simulink library "TriadActivation_lib"  (R2018b)
settings: Solver=VariableStepAuto  StartTime=0.0  StopTime=10.0  RelTol=1e-3
undefined symbols (not defined in the file): fswParams
libraries: dspswit3 x1
settings Model: Creator=kylle  LastModifiedBy=kylle

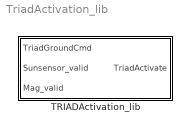
== system TriadActivation_lib ==
  TRIADActivation_lib : Subsystem  TreatAsAtomicUnit=on
      settings: RTWFcnNameOpts=Use subsystem name  RTWFileNameOpts=Use subsystem name

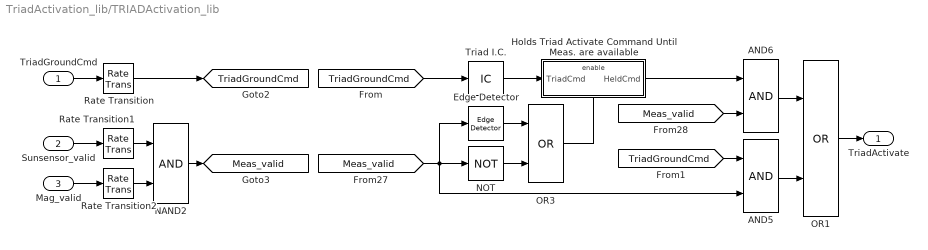
== system TriadActivation_lib/TRIADActivation_lib ==
  TriadGroundCmd : Inport
  Sunsensor_valid : Inport  Port=2
  Mag_valid : Inport  Port=3
  AND5 : Logic  AllPortsSameDT=off  OutDataTypeStr=boolean
  AND6 : Logic  AllPortsSameDT=off  OutDataTypeStr=boolean
  Edge Detector : dspswit3/Edge Detector  InputProcessing=Columns as channels (frame based)
      settings: SourceProductName=DSP System Toolbox  SourceProductBaseCode=DS
  Holds Triad Activate Command Until Meas. are available : Subsystem  TreatAsAtomicUnit=on
  NAND2 : Logic  AllPortsSameDT=off  OutDataTypeStr=boolean
  NOT : Logic  Operator=NOT  AllPortsSameDT=off  OutDataTypeStr=boolean
  OR1 : Logic  Operator=OR  AllPortsSameDT=off  OutDataTypeStr=boolean
  OR3 : Logic  Operator=OR  AllPortsSameDT=off  OutDataTypeStr=boolean
  Rate Transition : RateTransition  InitialCondition=fswParams.estimation.ic.activate_triad  OutPortSampleTime=fswParams.sample_time_s
  Rate Transition1 : RateTransition  OutPortSampleTime=fswParams.sample_time_s
  Rate Transition2 : RateTransition  OutPortSampleTime=fswParams.sample_time_s
  Triad I.C. : InitialCondition  Value=fswParams.estimation.ic.activate_triad
  TriadActivate : Outport
  tag scope: Meas_valid=global, TriadGroundCmd=global
  wires:
  [Meas_valid] -> AND6/2
  Holds Triad Activate Command Until Meas. are available/1(HeldCmd) -> AND6/1
  AND5/1 -> OR1/2
  AND6/1 -> OR1/1
  [Meas_valid] -> Edge Detector/1, NOT/1, AND5/2
  NAND2/1 -> [Meas_valid]
  OR3/1 -> Holds Triad Activate Command Until Meas. are available/Enable
  NOT/1 -> OR3/2
  Triad I.C./1 -> Holds Triad Activate Command Until Meas. are available/1(TriadCmd)
  Edge Detector/1 -> OR3/1
  Rate Transition2/1 -> NAND2/2
  Rate Transition1/1 -> NAND2/1
  [TriadGroundCmd] -> AND5/1
  Mag_valid/1 -> Rate Transition2/1
  Sunsensor_valid/1 -> Rate Transition1/1
  OR1/1 -> TriadActivate/1
  TriadGroundCmd/1 -> Rate Transition/1
  Rate Transition/1 -> [TriadGroundCmd]
  [TriadGroundCmd] -> Triad I.C./1

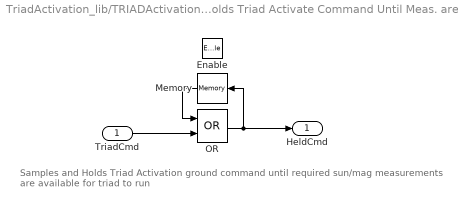
== system TriadActivation_lib/TRIADActivation_lib/Holds Triad Activate Command Until Meas. are available ==
  note: Samples and Holds Triad Activation ground command until required sun/mag measurements are available for triad to run
  TriadCmd : Inport
  Enable : EnablePort  StatesWhenEnabling=reset
  Memory : Memory
  OR : Logic  Operator=OR  AllPortsSameDT=off  OutDataTypeStr=boolean
  HeldCmd : Outport  OutputWhenDisabled=reset  InitialOutput=[0]
  wires:
  OR/1 -> HeldCmd/1, Memory/1
  Memory/1 -> OR/1
  TriadCmd/1 -> OR/2
